simulink model "project_2023_11_6_p91"  (R2017b)
settings: Solver=VariableStepAuto  StartTime=0.0  StopTime=100  RelTol=1e-3
settings Model: Creator=Administrator  LastModifiedBy=Administrator

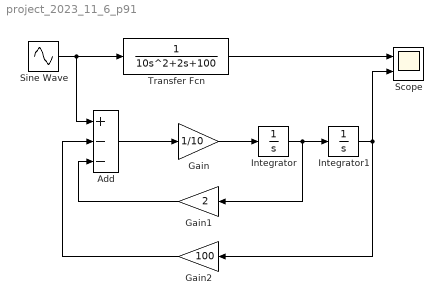
== system project_2023_11_6_p91 ==
  Add : Sum  Inputs=+--
  Gain : Gain  Gain=1/10
  Gain1 : Gain  Gain=2
  Gain2 : Gain  Gain=100
  Integrator : Integrator
  Integrator1 : Integrator
  Scope : Scope  NumInputPorts=2
  Sine Wave : Sin  SampleTime=0
  Transfer Fcn : TransferFcn  Denominator=[10 2 100]
  wires:
  Sine Wave/1 -> Transfer Fcn/1, Add/1
  Gain1/1 -> Add/3
  Gain2/1 -> Add/2
  Transfer Fcn/1 -> Scope/1
  Integrator1/1 -> Gain2/1, Scope/2
  Integrator/1 -> Integrator1/1, Gain1/1
  Gain/1 -> Integrator/1
  Add/1 -> Gain/1
